simulink model "HW5_b"  (R2024b)
settings: Solver=VariableStepAuto  StartTime=0.0  StopTime=50  RelTol=1e-3
settings Model: Creator=patrickstar  LastModifiedBy=patrickstar

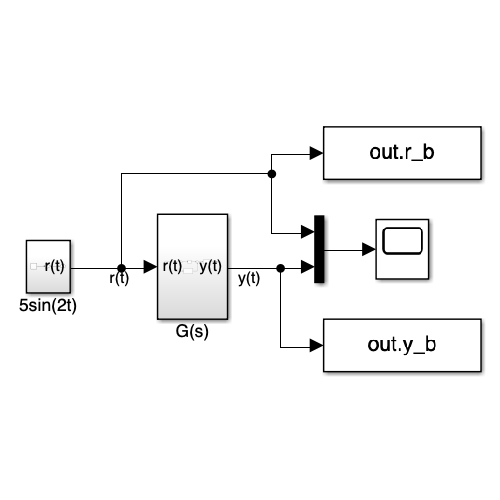
[thumbnail: Simulink's stored preview of the top-level diagram]
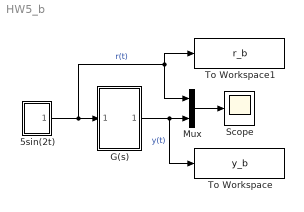
== system HW5_b ==
  5sin(2t) : Subsystem
  G(s) : Subsystem
  Mux : Mux  Inputs=2
  Scope : Scope
  To Workspace : ToWorkspace  VariableName=y_b  SaveFormat=Timeseries  SampleTime=-1
  To Workspace1 : ToWorkspace  VariableName=r_b  SaveFormat=Timeseries  SampleTime=-1
  wires:
  5sin(2t)/1(r(t)) -> Mux/1, To Workspace1/1, G(s)/1(r(t))  "r(t)"
  Mux/1 -> Scope/1
  G(s)/1(y(t)) -> To Workspace/1, Mux/2  "y(t)"

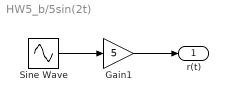
== system HW5_b/5sin(2t) ==
  Gain1 : Gain  Gain=5
  Sine Wave : Sin  Frequency=2  SampleTime=0
  r(t) : Outport
  wires:
  Gain1/1 -> r(t)/1
  Sine Wave/1 -> Gain1/1

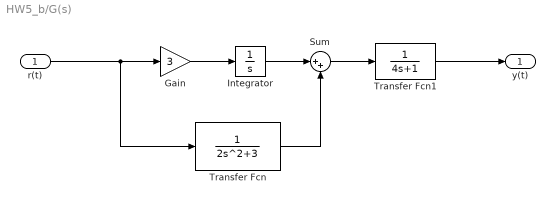
== system HW5_b/G(s) ==
  r(t) : Inport
  Gain : Gain  Gain=3
  Integrator : Integrator
  Sum : Sum  Inputs=|++
  Transfer Fcn : TransferFcn  Denominator=[2 0 3]
  Transfer Fcn1 : TransferFcn  Denominator=[4 1]
  y(t) : Outport
  wires:
  Transfer Fcn/1 -> Sum/2
  r(t)/1 -> Transfer Fcn/1, Gain/1
  Sum/1 -> Transfer Fcn1/1
  Integrator/1 -> Sum/1
  Transfer Fcn1/1 -> y(t)/1
  Gain/1 -> Integrator/1
